simulink model "SynchronousMachine"  (R2023b)
settings: Solver=VariableStepAuto  StartTime=0.0  StopTime=32  MaxStep=0.004  RelTol=1e-8
undefined symbols (not defined in the file or in its folder): Continuous, D1, Delta, spsHTGModel
libraries: simulink_extras x3, spsThreePhaseParallelRLCLoadLib x2, spsLoadFlowBusLib x2, spsThreePhaseSourceLib x1, spsThreePhaseFaultLib x1, spsExcitationSystemLib x1, slpidlib x1, eeSmST4C x1, SignalEditorBlockLib x1, spsSynchronousMachinepuStandardLib x1, spsThreePhaseTransformerTwoWindingsLib x1, spspowerguiLib x1
settings Model: SimulationMode=accelerator  Creator=The MathWorks, Inc.  LastModifiedBy=qweuror
settings SolverCC: AlgebraicLoopSolver=TrustRegion
settings DataIOCC: SaveFormat=Array  SignalLoggingName=sigsOut
settings OptimizationCC: BlockReduction=off  BooleanDataType=off  ExpressionDepthLimit=2147483647  InitFltsAndDblsToZero=on  EfficientMapNaN2IntZero=off  LifeSpan=inf
settings DebuggingCC: UnderspecifiedInitializationDetection=Classic  MergeDetectMultiDrivingBlocksExec=none  CheckExecutionContextPreStartOutputMsg=on  SignalResolutionControl=TryResolveAllWithWarning  MultiTaskDSMMsg=warning  MultiTaskCondExecSysMsg=none  SigSpecEnsureSampleTimeMsg=none  FcnCallInpInsideContextMsg=warning  StateNameClashWarn=warning  SFUnexpectedBacktrackingDiag=warning  SFNoUnconditionalDefaultTransitionDiag=warning  SFExecutionAtInitializationDiag=none  ArithmeticOperatorsInVariantConditions=warning
settings HardwareCC: ProdBitPerPointer=32  ProdBitPerSizeT=32  ProdBitPerPtrDiffT=32  ProdLargestAtomicFloat=None  ProdIntDivRoundTo=Undefined  ProdEndianess=Unspecified  ProdWordSize=32  ProdHWDeviceType=32-bit Generic  TargetUnknown=on
settings ModelReferenceCC: EnableRefExpFcnMdlSchedulingChecks=on  PropagateSignalLabelsOutOfModel=off
settings SFSimCC: SimUseLocalCustomCode=off  CustomCodeUndefinedFunction=UseInterfaceOnly
settings RTWCC: RTWUseLocalCustomCode=off  DLArmComputeVersion=19.05
settings CodeAppCC: StateflowObjectComments=on
settings GRTTargetCC: TargetLangStandard=C89/C90 (ANSI)  CombineOutputUpdateFcns=off  GRTInterface=on
settings ConfigComp: CovMetricSettings=dw  CovSaveCumulativeToWorkspaceVar=on  CovSaveSingleToWorkspaceVar=on  CovExternalEMLEnable=off  CovSFcnEnable=off
settings SimscapeCC: SimscapeNormalizeSystem=off

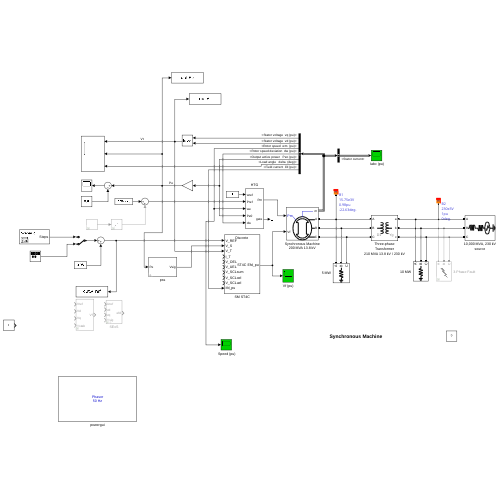
[thumbnail: Simulink's stored preview of the top-level diagram]
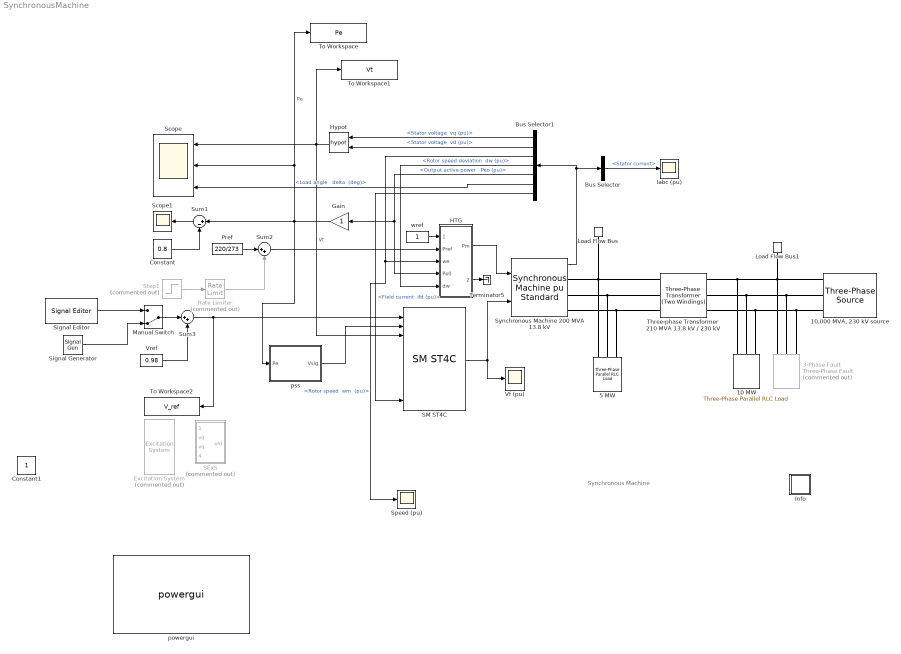
== system SynchronousMachine ==
  note: Synchronous Machine
  " Iabc (pu)" : Scope
  " Speed (pu)" : Scope
  10 MW : spsThreePhaseParallelRLCLoadLib/Three-Phase Parallel RLC Load  LConnTagsString=A|B|C  Configuration=Y (grounded)  NominalVoltage=230e3  Vabc=[1e3 1e3 1e3]  Vabcp=[1e3 1e3 1e3]  NominalFrequency=50  UnbalancedPower=off  ActivePower=10000000  InductivePower=0  CapacitivePower=0  Pabc=[10e3 9e3 11e3]  QLabc=[100 90 110]  QCabc=[100 90 110]  Pabcp=[10e3 9e3 11e3]  QLabcp=[100 90 110]  QCabcp=[100 90 110]  Measurements=None  LoadType=constant Z
  "10,000 MVA, 230 kV source" : spsThreePhaseSourceLib/Three-Phase Source  InternalConnection=Yg  VoltagePhases=off  Voltage=(230000)*1.00373  PhaseAngle=-1.1862  Voltage_phases=[25e3 25e3 25e3]/sqrt(3)  PhaseAngles_phases=[0 -120 +120]  Frequency=50  NonIdealSource=on  SpecifyImpedance=on  Resistance=0.529  Inductance=0.0140  ShortCircuitLevel=10000e6  BaseVoltage=230e3  XRratio=10  BusType=swing  Pref=0  Qref=0  Prefabc=[10e3, 10e3, 10e3]  Qrefabc=[0, 0, 0]  Qmin=-Inf  Qmax=Inf
  3-Phase Fault : spsThreePhaseFaultLib/Three-Phase Fault  Commented=on  InitialStates=0  FaultA=on  FaultB=on  FaultC=on  GroundFault=on  SwitchTimes=[ 0.1 0.924]  External=off  SwitchStatus=NaN  FaultResistance=1e-3  GroundResistance=1e-3  SnubberResistance=inf  SnubberCapacitance=inf  Measurements=None
  5 MW : spsThreePhaseParallelRLCLoadLib/Three-Phase Parallel RLC Load  LConnTagsString=A|B|C  Configuration=Y (grounded)  NominalVoltage=13.8e3  Vabc=[1e3 1e3 1e3]  Vabcp=[1e3 1e3 1e3]  NominalFrequency=50  UnbalancedPower=off  ActivePower=5000000  InductivePower=0  CapacitivePower=0  Pabc=[10e3 9e3 11e3]  QLabc=[100 90 110]  QCabc=[100 90 110]  Pabcp=[10e3 9e3 11e3]  QLabcp=[100 90 110]  QCabcp=[100 90 110]  Measurements=None  LoadType=constant Z
  Bus Selector : BusSelector  OutputSignals=Stator current
  Bus Selector1 : BusSelector  OutputSignals="dq0 components.Stator voltage  vq (pu),dq0 components.Stator voltage  vd (pu),Mechanical.Rotor speed  wm  (pu),Mechanical.Rotor speed deviation  dw (pu),Output active power   Peo (pu),Load angle   delta  (deg),dq0 components.Field current  ifd (pu)"
  Constant : Constant  Value=0.8
  Constant1 : Constant
  Excitation System : spsExcitationSystemLib/Excitation System  Commented=on  tr=20e-3  reg=[300 0.001]  exc=[ 1, 0 ]  tgr=[0.5 0.1]  damp=[ 0.002, 0.1 ]  sat=[ 0, 0 ]  lim=[ -11.5, 11.5, 0 ]  v0=[0.98 1.1855]
  Gain : Gain
  HTG : Subsystem  AncestorBlock=spsHydraulicTurbineandGovernorLib/Hydraulic Turbine and Governor  DialogController=POWERSYS.PowerSysDialog  mask(Hydraulic Turbine and Governor){sm=[ 10/3  0.07 ], gate=[  0.01  0.97518  -0.1  0.1 ], reg=[0.05 0.01 0.23997301034918 0 0.01], hyd=[  0  2.67  ], dref=0, po=0.80696}
      mask prompts: sm "Servo-motor [ Ka()  Ta(sec) ]:"; gate "Gate opening limits [ gmin,gmax(pu)    vgmin,vgmax(pu/s) ]:"; reg "Permanent droop and regulator  [ Rp() Kp() Ki() Kd() Td(s) ]:"; hyd "Hydraulic turbine [ beta()  Tw(sec) ]:"; dref "Droop reference (0=power error, 1=gate opening):"; po "Initial mechanical power (pu):"
      mask help: Implements a hydraulic turbine combined to a PID governor system.
      mask init:
      | block = gcb;
      | [Ts, WantBlockChoice,ka,ta,gmin,gmax,vgmin,vgmax,Rp,Kp,ki,kd,td,beta,tw,go] = powericon('HydraulicTurbineInit',block,sm,gate,reg,hyd,po);
      | powericon('SetInternalModels','set',block,WantBlockChoice);
      settings: OpenFcn=sps_rtmsupport('OpenFcn',gcbh)
      mask Help: helpview(psbhelp);
      mask Display: disp('')
  Hypot : Math  Operator=hypot
  Info : Subsystem
      settings: OpenFcn="showExample(\"simscapeelectricalsps/SynchronousMachineExample\")"
      mask Display: disp('?')
  Load Flow Bus : spsLoadFlowBusLib/Load Flow Bus  LConnTagsString=a  Phases=single  Connectors=on one side  ID=B1  Vbase=15.75e3  Vref=0.98  Vangle=0  VLF=0.98  VLFb=1  VLFc=1  angleLF=-22.63  angleLFb=0  angleLFc=0
      settings: AttributesFormatString=%<ID>\n%<Vbase>V\n%<VLF>pu\n%<angleLF>deg.
  Load Flow Bus1 : spsLoadFlowBusLib/Load Flow Bus  LConnTagsString=a  Phases=single  Connectors=on one side  ID=B2  Vbase=230e3  Vref=1  Vangle=0  VLF=1  VLFb=1  VLFc=1  angleLF=0  angleLFb=0  angleLFc=0
      settings: AttributesFormatString=%<ID>\n%<Vbase>V\n%<VLF>pu\n%<angleLF>deg.
  Manual Switch : ManualSwitch  CurrentSetting=0
  Pref : Constant  Value=220/273
  Rate Limiter : RateLimiter  Commented=on  RisingSlewLimit=(12.4/200)/60  FallingSlewLimit=-(12.4/200)/60  SampleTimeMode=inherited  InitialCondition=220/273
  SExS : Subsystem  Commented=on  mask{Kp=6, Ki=12, Ke=3, Te=0.02, Efdmax=5, Efdmin=-4, Vf0=1.98039}
  SM ST4C : eeSmST4C/SM ST4C  E_FD0=1.61651  V_T0=1  I_T0=1  Ts=0.004  R_C=0  X_C=0  T_R=0  K_PR=10.75  K_IR=10.75  T_A=0.02  V_Rmax=1  V_Rmin=-0.87  K_PM=1  K_IM=0  V_Mmax=99  V_Mmin=-99  V_Amax=99  V_Amin=-99  K_G=0  T_G=0  V_Gmax=99  vsInputLocation=Summation point before take-over UEL  oelInputLocation=Unused  uelInputLocation=Unused  sclInputLocation=Unused  K_C=0.113  K_P=5.2  K_I=0  X_L=0  theta_P=0  V_Bmax=11.63  SW1=Position A: power source derived from generator terminal voltage
      settings: LibrarySourceBlock=ee_sl_lib/SM Control/SM ST4C
  Scope : Scope  NumInputPorts=3
  Scope1 : Scope
  Signal Editor : SignalEditorBlockLib/Signal Editor  FileName=steps.mat  ActiveScenario=Scenario  ActiveSignal=Steps  IsBus=off  OutputBusObjectStr=Bus: BusObject  SampleTime=0  Interpolate=off  ZeroCross=off  OutputAfterFinalValue=Setting to zero  Unit=inherit  PreserveSignalName=on  ApplySigPropsToAllScenarios=on  ApplySigPropsToAllSignals=off
  Signal Generator : SignalGenerator  Amplitude=0.01  Frequency=5.5
  Step1 : Step  Commented=on  Time=10  After=0.05  SampleTime=0
  Sum1 : Sum  Inputs=|+-
  Sum2 : Sum  Inputs=|++
  Sum3 : Sum  Inputs=|++
  Synchronous Machine 200 MVA 13.8 kV : spsSynchronousMachinepuStandardLib/Synchronous Machine pu Standard  PresetModel=No  MechanicalLoad=Mechanical power Pm  ShowDetailedParameters=on  RotorType=Round  Units=per unit standard parameters  MeasurementBus=off  NominalParameters="[ 273E6  15.75e3   50 ]"  Reactances1=[ 1.7 0.245 0.185 1.62 0.256 0.155 0.147 ]  Reactances2=[ 1.305, 0.296, 0.252, 0.474, 0.243, 0.18 ]  dAxisTimeConstants=Open-circuit  qAxisTimeConstants=Open-circuit  TimeConstants1=[]  TimeConstants2=[4.8 0.023 0.5 0.02]  TimeConstants3=[]  TimeConstants4=[]  TimeConstants5=[ 1.01, 0.053, 0.1 ]  TimeConstants6=[]  TimeConstants7=[]  TimeConstants8=[]  StatorResistance=0.0016  Mechanical=[ 4.56 0 2]  PolePairs=2  InitialConditions=[0 -54.259 0.82828 0.82828 0.82828 -15.7481 -135.748 104.252 1.61651]  SetSaturation=off  Saturation=[0.6404,0.7127,0.8441,0.9214,0.9956,1.082,1.19,1.316,1.457;0.7,0.7698,0.8872,0.9466,0.9969,1.046,1.1,1.151,1.201]  LoadFlowParameters=[1 150000000 0 0]  TsPowergui=0  TsBlock=-1  IterativeModel=Trapezoidal non iterative  IterativeDiscreteModel=Trapezoidal non iterative  BusType=PV  Pref=220000000  Qref=0  Qmin=-Inf  Qmax=Inf  PLF=0  QLF=0
  Terminator5 : Terminator
  Three-phase Transformer 210 MVA 13.8 kV / 230 kV : spsThreePhaseTransformerTwoWindingsLib/Three-Phase Transformer (Two Windings)  Winding1Connection=Delta (D1)  Winding2Connection=Yg  CoreType=Three single-phase transformers  SetSaturation=off  Hysteresis=off  DataFile='hysteresis'  SetInitialFlux=off  Measurements=None  UNITS=pu  NominalPower=[ 273e6 50 ]  Winding1="[ 15.75e3 0.0027  0.08]"  Winding2=[ 230e3 0.0027 0.08]  Rm=500  Lm=500  L0=0.5  Saturation="[ 0,0  ;  0.005,1.2  ;  1.0,1.4 ]"  InitialFluxes=[ 0.8 , -0.8 , 0.7 ]  BreakLoop=off  DiscreteSolver=Trapezoidal iterative  DataType=off  TransfoNumber=0
  To Workspace : ToWorkspace  VariableName=Pe  SaveFormat=Timeseries  SampleTime=-1
  To Workspace1 : ToWorkspace  VariableName=Vt  SaveFormat=Timeseries  SampleTime=-1
  To Workspace2 : ToWorkspace  VariableName=V_ref  SaveFormat=Timeseries  SampleTime=-1
  Vf (pu) : Scope
  Vref : Constant  Value=0.98
  powergui : spspowerguiLib/powergui  Priority=2  SimulationMode=Phasor  SampleTime=0  frequency=50  Iterations=50  frequencyindice=50  Pbase=100e6  ErrMax=0.0001  UnitsV=kV  UnitsW=MW  buscounter=0  FunctionMessages=off  echomessages=off  EnableUseOfTLC=off  CurrentSourceSwitches=off  DisableSnubberDevices=off  DisableRonSwitches=off  DisableVfSwitches=off  DisplayEquations=off  AutomaticDiscreteSolvers=off  SolverType=Tustin  Interpol=off  ExternalGateDelay=off  methode=off  Ts=0  x0status=blocks  SPID=on  SwTol=0  HookPort=off  NonlinearTolerance=1e-4  nMaxIteration=100  ContinueOnMaxIteration=off  RestoreLinks=warning  ResistiveCurrentMeasurement=off  Frange=logspace(0,3,50)  Ylog=off  Xlog=off  ShowGrid=off  save=off  variable=ZData  structure=0  ZoomFFT=on  StartTime=0.0  cycles=2  DisplayStyle=off  fundamental=60  FreqAxis=off  MaxFrequency=1000  frequencyindicesteady=1  RmsSteady=1  display=off
  pss : Subsystem  mask{T1=0.01, T2=0.27729, Kpe=0.093962, Pe0=220/273}
  wref : Constant
  wires:
  HTG/2(gate) -> Terminator5/1
  Vref/1 -> Sum3/2
  Pref/1 -> Sum2/1
  wref/1 -> HTG/1(wref)
  SM ST4C/1 -> Synchronous Machine 200 MVA 13.8 kV/2, Vf (pu)/1
  HTG/1(Pm) -> Synchronous Machine 200 MVA 13.8 kV/1
  Synchronous Machine 200 MVA 13.8 kV/1 -> Bus Selector/1, Bus Selector1/1
  Bus Selector/1 -> " Iabc (pu)"/1  "<Stator current>"
  Bus Selector1/1 -> Hypot/1  "<Stator voltage  vq (pu)>"
  Bus Selector1/2 -> Hypot/2  "<Stator voltage  vd (pu)>"
  Bus Selector1/3 -> HTG/3(we), " Speed (pu)"/1  "<Rotor speed  wm  (pu)>"
  Bus Selector1/4 -> HTG/5(dw)  "<Rotor speed deviation  dw (pu)>"
  Bus Selector1/5 -> HTG/4(Pe0), Gain/1  "<Output active power   Peo (pu)>"
  Hypot/1 -> To Workspace1/1, SM ST4C/3, Scope/1  "Vt"
  Gain/1 -> To Workspace/1, Scope/2, Sum1/1, pss/1(Pe)  "Pe"
  Bus Selector1/6 -> Scope/3  "<Load angle   delta  (deg)>"
  Signal Generator/1 -> Manual Switch/2
  Sum1/1 -> Scope1/1
  Constant/1 -> Sum1/2
  Sum2/1 -> HTG/2(Pref)
  Step1/1 -> Rate Limiter/1
  pss/1(Vsig) -> SM ST4C/2
  Bus Selector1/7 -> SM ST4C/10  "<Field current  ifd (pu)>"
  Rate Limiter/1 -> Sum2/2
  Signal Editor/1 -> Manual Switch/1
  Manual Switch/1 -> Sum3/1
  Sum3/1 -> To Workspace2/1, SM ST4C/1
  connections:
  Synchronous Machine 200 MVA 13.8 kV/RConn3 -- 5 MW/LConn3 -- Three-phase Transformer 210 MVA 13.8 kV / 230 kV/LConn3
  Synchronous Machine 200 MVA 13.8 kV/RConn2 -- 5 MW/LConn2 -- Three-phase Transformer 210 MVA 13.8 kV / 230 kV/LConn2
  Synchronous Machine 200 MVA 13.8 kV/RConn1 -- 5 MW/LConn1 -- Three-phase Transformer 210 MVA 13.8 kV / 230 kV/LConn1 -- Load Flow Bus/LConn1
  Three-phase Transformer 210 MVA 13.8 kV / 230 kV/RConn1 -- 3-Phase Fault/LConn1 -- "10,000 MVA, 230 kV source"/RConn1 -- Load Flow Bus1/LConn1 -- 10 MW/LConn1
  Three-phase Transformer 210 MVA 13.8 kV / 230 kV/RConn2 -- 3-Phase Fault/LConn2 -- "10,000 MVA, 230 kV source"/RConn2 -- 10 MW/LConn2
  Three-phase Transformer 210 MVA 13.8 kV / 230 kV/RConn3 -- 3-Phase Fault/LConn3 -- "10,000 MVA, 230 kV source"/RConn3 -- 10 MW/LConn3

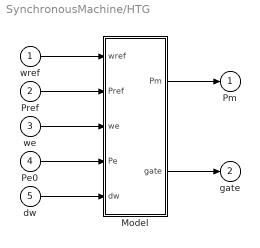
== system SynchronousMachine/HTG ==
  wref : Inport
  Pref : Inport  Port=2
  we : Inport  Port=3
  Pe0 : Inport  Port=4
  dw : Inport  Port=5
  Model : Subsystem  AncestorBlock=spsHTGModel/Continuous  mask(Hydraulic Turbine and Governor){sm=sm, gate=gate, reg=reg, hyd=hyd, dref=dref, po=po}
      mask prompts: sm "Servo-motor [ Ka()  Ta(sec) ]:"; gate "Gate opening limits [ gmin,gmax(pu)    vgmin,vgmax(pu/s) ]:"; reg "Permanent droop and regulator  [ Rp() Kp() Ki() Kd() Td(s) ]:"; hyd "Hydraulic turbine [ beta()  Tw(sec) ]:"; dref "Droop reference (0=power error, 1=gate opening):"; po "Initial mechanical power (pu):"
      mask help:
      | Implements a hydraulic turbine combined to a PID governor system.
      |
      | 1st input: desired speed (p.u.);
      | 2nd input: desired electrical power (p.u.);
      | 3rd input: synchronous machine's actual speed (p.u., measurement output 13 of SM block);
      | 4th input: synchronous machine's actual electrical power (p.u., measurement output 14 of SM block);
      | 5th input: synchronous machine's actual speed deviation with respect to nominal (%, measurement output 15 of SM block);
      |
      | 1st output: mechanical power to be applied to the Synchronous Machine block's 1st input (p.u.);
      | 2nd output: gate opening (p.u.).
      mask init:
      | ka=sm(1);ta=sm(2);gmin=gate(1);gmax=gate(2);vgmin=gate(3);vgmax=gate(4);Rp=reg(1);kp=reg(2);ki=reg(3);kd=reg(4);td=reg(5);beta=hyd(1);tw=hyd(2);go=po*(gmax-gmin);
      mask Help: helpview(psbhelp);
  Pm : Outport  InitialOutput=0  VectorParamsAs1DForOutWhenUnconnected=off
  gate : Outport  Port=2  InitialOutput=0  VectorParamsAs1DForOutWhenUnconnected=off
  wires:
  wref/1 -> Model/1(wref)
  Pref/1 -> Model/2(Pref)
  we/1 -> Model/3(we)
  Pe0/1 -> Model/4(Pe)
  dw/1 -> Model/5(dw)
  Model/2(gate) -> gate/1
  Model/1(Pm) -> Pm/1

== system SynchronousMachine/Info ==

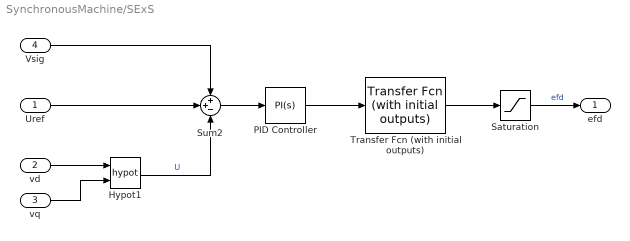
== system SynchronousMachine/SExS ==
  Uref : Inport
  vd : Inport  Port=2
  vq : Inport  Port=3
  Vsig : Inport  Port=4
  Hypot1 : Math  Operator=hypot
  PID Controller : slpidlib/PID Controller  Controller=PI  Form=Parallel  TimeDomain=Continuous-time  UseExternalTs=off  SampleTime=-1  IntegratorMethod=Forward Euler  FilterMethod=Forward Euler  ControllerParametersSource=internal  P=Kp  I=Ki  UseKiTs=off  D=0  N=100  UseFilter=on  TunerSelectOption=Transfer Function Based (PID Tuner App)  InitialConditionSource=internal  InitialConditionForIntegrator=Vf0/Ke  InitialConditionForFilter=0  DifferentiatorICPrevScaledInput=0  ExternalReset=none  TrackingMode=off  Kt=1  LimitOutput=off  SatLimitsSource=internal  UpperSaturationLimit=inf  LowerSaturationLimit=-inf  LinearizeAsGain=on  AntiWindupMode=none  Kb=1  LimitIntegrator=off  UpperIntegratorSaturationLimit=inf  LowerIntegratorSaturationLimit=-inf  POutMin=[]  POutMax=[]  IOutMin=[]  IOutMax=[]  DOutMin=[]  DOutMax=[]  NOutMin=[]  NOutMax=[]  SumOutMin=[]  SumOutMax=[]  SaturationOutMin=[]  SaturationOutMax=[]  PParamMin=[]  PParamMax=[]  IParamMin=[]  IParamMax=[]  DParamMin=[]  DParamMax=[]  NParamMin=[]  NParamMax=[]  KbParamMin=[]  KbParamMax=[]  KtParamMin=[]  KtParamMax=[]  KbOutMin=[]  KbOutMax=[]  KtOutMin=[]  KtOutMax=[]  IntegratorOutMin=[]  IntegratorOutMax=[]  FilterOutMin=[]  FilterOutMax=[]  SumI1OutMin=[]  SumI1OutMax=[]  SumI2OutMin=[]  SumI2OutMax=[]  SumI3OutMin=[]  SumI3OutMax=[]  SumI4OutMin=[]  SumI4OutMax=[]  SumDOutMin=[]  SumDOutMax=[]  DifferentiatorOutMin=[]  DifferentiatorOutMax=[]  FilterDiffOutCoefMin=[]  FilterDiffOutCoefMax=[]  ReciprocalOutMin=[]  ReciprocalOutMax=[]  SumDenOutMin=[]  SumDenOutMax=[]  SumNumOutMin=[]  SumNumOutMax=[]  DivideOutMin=[]  DivideOutMax=[]  UdiffTsProdOutMin=[]  UdiffTsProdOutMax=[]  NTsProdOutMin=[]  NTsProdOutMax=[]  UintegralTsProdOutMin=[]  UintegralTsProdOutMax=[]  UngainTsProdOutMin=[]  UngainTsProdOutMax=[]  ClampingZeroOutDataTypeStr=Inherit: Inherit via back propagation  ClampingZeroOutMin=[]  ClampingZeroOutMax=[]  FilterDenConstantOutDataTypeStr=Inherit: Inherit via back propagation  FilterDenConstantOutMin=[]  FilterDenConstantOutMax=[]  PCopyOutDataTypeStr=Inherit: Inherit via back propagation  PCopyOutMin=[]  PCopyOutMax=[]  NCopyOutDataTypeStr=Inherit: Inherit via back propagation  NCopyOutMin=[]  NCopyOutMax=[]  IntegratorContinuousStateAttributes=''  IntegratorStateMustResolveToSignalObject=off  IntegratorRTWStateStorageClass=Auto  FilterContinuousStateAttributes=''  FilterStateMustResolveToSignalObject=off  FilterRTWStateStorageClass=Auto  ParallelPVariant=InternalParameters  IdealPVariant=Disabled  IVariant=InternalParameters  DVariant=Disabled  IntegratorVariant=Continuous  SatVariant=Disabled  AWVariant=Passthrough  PCopyVariant=Disabled  TRVariant=Disabled  FdbkBlocksVariant=Forward  IdealPFdbkVariant=Disabled  SatFdbkVariant=Disabled  DerivativeFilterVariant=Disabled  NVariant=Disabled  NCopyVariant=Disabled_SignalSpec  FilterICVariant=Disabled  IntegratorICVariant=InternalICs  ExternalResetVariant=Disabled  TRSumVariant=Passthrough  SumFdbkVariant=Disabled  SumVariant=Sum_PI  TsampFilterVariant=InternalTs  TsampNgainVariant=Passthrough  TsampIntegralVariant=Disabled_SignalSpec  ExternalSaturationOutDataTypeStr=Inherit: Same as second input
  Saturation : Saturate  UpperLimit=Efdmax  LowerLimit=Efdmin
  Sum2 : Sum  Inputs=++-
  Transfer Fcn (with initial outputs) : simulink_extras/Additional Linear/Transfer Fcn (with initial outputs)  N=[Ke]  D=[Te 1]  Y0=Vf0  U0=Vf0/Ke
  efd : Outport
  wires:
  Uref/1 -> Sum2/2
  Transfer Fcn (with initial outputs)/1 -> Saturation/1
  Sum2/1 -> PID Controller/1
  PID Controller/1 -> Transfer Fcn (with initial outputs)/1
  vq/1 -> Hypot1/2
  vd/1 -> Hypot1/1
  Saturation/1 -> efd/1  "efd"
  Hypot1/1 -> Sum2/3  "U"
  Vsig/1 -> Sum2/1

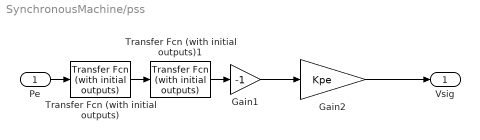
== system SynchronousMachine/pss ==
  Pe : Inport
  Gain1 : Gain  Gain=-1
  Gain2 : Gain  Gain=Kpe
  Transfer Fcn (with initial outputs) : simulink_extras/Additional Linear/Transfer Fcn (with initial outputs)  N=[1]  D="[T1  1]"  Y0=Pe0  U0=Pe0
  Transfer Fcn (with initial outputs)1 : simulink_extras/Additional Linear/Transfer Fcn (with initial outputs)  N=[T2 0]  D="[T2  1]"  Y0=0  U0=Pe0
  Vsig : Outport
  wires:
  Transfer Fcn (with initial outputs)1/1 -> Gain1/1
  Gain1/1 -> Gain2/1
  Pe/1 -> Transfer Fcn (with initial outputs)/1
  Transfer Fcn (with initial outputs)/1 -> Transfer Fcn (with initial outputs)1/1
  Gain2/1 -> Vsig/1

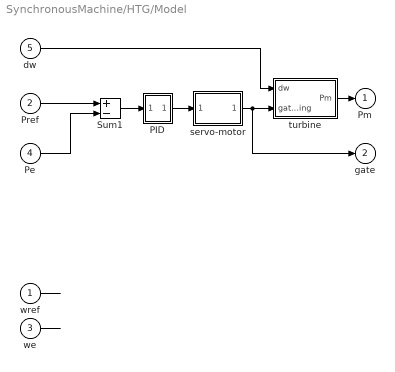
== system SynchronousMachine/HTG/Model ==
  wref : Inport
  Pref : Inport  Port=2
  we : Inport  Port=3
  Pe : Inport  Port=4
  dw : Inport  Port=5
  PID : Subsystem  mask(PID(2) Controller){}
      mask Display: disp('PID')
  Sum1 : Sum  Inputs=+-  InputSameDT=on  SaturateOnIntegerOverflow=on  OutDataTypeStr=Inherit: Same as first input
  servo-motor : Subsystem
      mask Display: disp('servo-\nmotor')
  turbine : Subsystem
      mask Display: disp('hydraulic\nturbine')
  Pm : Outport  InitialOutput=0
  gate : Outport  Port=2  InitialOutput=0
  wires:
  Sum1/1 -> PID/1(error)
  Pref/1 -> Sum1/1
  PID/1(Output) -> servo-motor/1(regulator's output)
  wref/1 -> ?
  we/1 -> ?
  servo-motor/1(gate opening) -> gate/1, turbine/2(gate opening)
  dw/1 -> turbine/1(dw)
  turbine/1(Pm) -> Pm/1
  Pe/1 -> Sum1/2

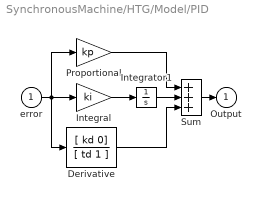
== system SynchronousMachine/HTG/Model/PID ==
  error : Inport
  Derivative : TransferFcn  Numerator=[ kd 0]  Denominator=[ td 1 ]
  Integral : Gain  Gain=ki  SaturateOnIntegerOverflow=on  OutDataTypeStr=Inherit: Same as input  ParamDataTypeStr=Inherit: Same as input
  Integrator1 : Integrator  InitialCondition=go
  Proportional : Gain  Gain=kp  SaturateOnIntegerOverflow=on  OutDataTypeStr=Inherit: Same as input  ParamDataTypeStr=Inherit: Same as input
  Sum : Sum  Inputs=+++  InputSameDT=on  SaturateOnIntegerOverflow=on  OutDataTypeStr=Inherit: Same as first input
  Output : Outport  InitialOutput=0
  wires:
  Integrator1/1 -> Sum/2
  Integral/1 -> Integrator1/1
  error/1 -> Proportional/1, Derivative/1, Integral/1
  Sum/1 -> Output/1
  Derivative/1 -> Sum/3
  Proportional/1 -> Sum/1

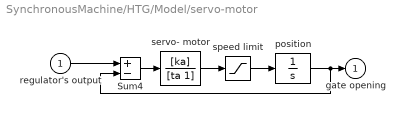
== system SynchronousMachine/HTG/Model/servo-motor ==
  regulator's output : Inport
  Sum4 : Sum  Inputs=+-  InputSameDT=on  SaturateOnIntegerOverflow=on  OutDataTypeStr=Inherit: Same as first input
  position : Integrator  InitialCondition=go  LimitOutput=on  UpperSaturationLimit=gmax  LowerSaturationLimit=gmin
  servo- motor : TransferFcn  Numerator=[ka]  Denominator=[ta 1]
  speed limit : Saturate  UpperLimit=vgmax  LowerLimit=vgmin
  gate opening : Outport  InitialOutput=0
  wires:
  position/1 -> Sum4/2, gate opening/1
  speed limit/1 -> position/1
  servo- motor/1 -> speed limit/1
  Sum4/1 -> servo- motor/1
  regulator's output/1 -> Sum4/1

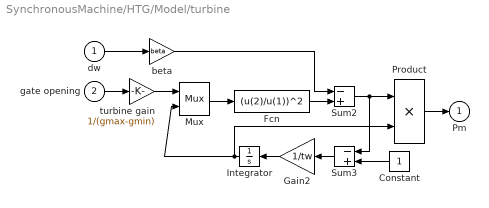
== system SynchronousMachine/HTG/Model/turbine ==
  dw : Inport
  gate opening : Inport  Port=2
  Constant : Constant
  Fcn : Fcn  Expr=(u(2)/u(1))^2
  Gain2 : Gain  Gain=1/tw  SaturateOnIntegerOverflow=on  OutDataTypeStr=Inherit: Same as input  ParamDataTypeStr=Inherit: Same as input
  Integrator : Integrator  InitialCondition=po
  Mux : Mux  Inputs=2
  Product : Product  InputSameDT=on  SaturateOnIntegerOverflow=on  OutDataTypeStr=Inherit: Same as first input
  Sum2 : Sum  Inputs=-+  InputSameDT=on  SaturateOnIntegerOverflow=on  OutDataTypeStr=Inherit: Same as first input
  Sum3 : Sum  Inputs=-+  InputSameDT=on  SaturateOnIntegerOverflow=on  OutDataTypeStr=Inherit: Same as first input
  beta : Gain  Gain=beta  SaturateOnIntegerOverflow=on  OutDataTypeStr=Inherit: Same as input  ParamDataTypeStr=Inherit: Same as input
  turbine gain : Gain  Gain=1/(gmax-gmin)  SaturateOnIntegerOverflow=on  OutDataTypeStr=Inherit: Same as input  ParamDataTypeStr=Inherit: Same as input
  Pm : Outport  InitialOutput=0
  wires:
  turbine gain/1 -> Mux/1
  gate opening/1 -> turbine gain/1
  Integrator/1 -> Product/2, Mux/2
  Mux/1 -> Fcn/1
  Fcn/1 -> Sum2/2
  Constant/1 -> Sum3/2
  Product/1 -> Pm/1
  Sum3/1 -> Gain2/1
  Gain2/1 -> Integrator/1
  Sum2/1 -> Sum3/1, Product/1
  beta/1 -> Sum2/1
  dw/1 -> beta/1
